simulink model "ModifiedSimulinkModel"  (R2016a)
settings: Solver=ode4  StartTime=0.0  StopTime=200  FixedStep=0.1  RelTol=1e-3
values from neighbouring files (symbols this model uses):
  engineblendfactormap = [0 0 0 0 0 0 0 0 0 0 0 0 ... (420 elements, 21x20)]    [blendfactorvariables.mat]
  motorblendfactormap = [1 1 1 1 1 1 1 1 1 1 1 1 ... (420 elements, 21x20)]    [blendfactorvariables.mat]
  v = [0 5 10 15 20 25 30 35 40 45 50 55 ... (21 elements, 1x21)]    [blendfactorvariables.mat]
  x = [0 1 2 3 4 5 6 7 8 9 10 11 ... (20 elements, 1x20)]    [blendfactorvariables.mat]
undefined symbols (not defined in the file or in its folder): sigbuilder_block
settings Model: Creator=Saumya Trivedi  LastModifiedBy=Saumya Trivedi

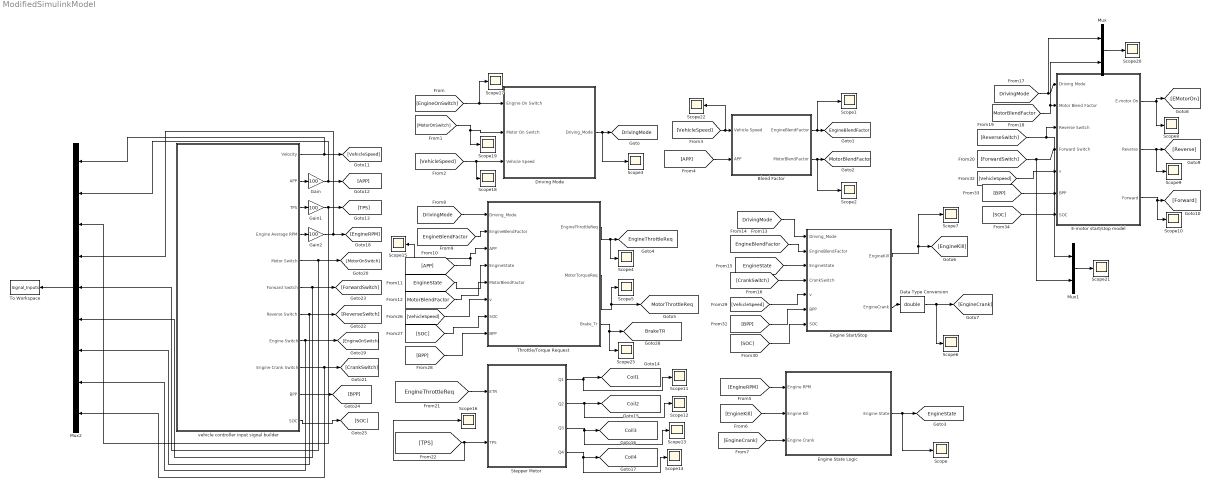
== system ModifiedSimulinkModel ==
  Blend Factor : Subsystem
  Data Type Conversion : DataTypeConversion  OutDataTypeStr=double
  Driving Mode : Subsystem
  E-motor start/stop model : Subsystem
  Engine Start/Stop : Subsystem
  Engine State Logic : Subsystem
  Gain : Gain  Gain=100
  Gain1 : Gain  Gain=100
  Gain2 : Gain  Gain=100
  Mux : Mux  Inputs=2
  Mux1 : Mux  Inputs=2
  Mux2 : Mux  Inputs=9
  Scope{,1..22,25} (24 alike) : Scope
  Stepper Motor : Subsystem
  Throttle/Torque Request : Subsystem
  To Workspace : ToWorkspace  VariableName=Signal_Inputs  SaveFormat=Structure With Time  SampleTime=-1
  vehicle controller input signal builder : Subsystem  Tag=STV Subsys  LoadFcn=sigbuilder_block('load');  StartFcn=sigbuilder_block('start');  StopFcn=sigbuilder_block('stop');  ClipboardFcn=sigbuilder_block('clipboard');  mask(Sigbuilder block){}
      mask help: Create and generate interchangeable groups of signals whose waveforms are piecewise linear.
      mask init:
      | if ~strcmp(get_param(bdroot(gcbh),'SimulationStatus'),'stopped') tuvar = sigbuilder_block('maskInit'); end
      settings: CopyFcn=sigbuilder_block('copy');  DeleteFcn=sigbuilder_block('delete');  ModelCloseFcn=sigbuilder_block('modelClose');  PreSaveFcn=sigbuilder_block('preSave');  PauseFcn=sigbuilder_block('pause')  ContinueFcn=sigbuilder_block('continue')  NameChangeFcn=sigbuilder_block('namechange');  OpenFcn=sigbuilder_block('open',[5.5 33.5 949 407 ]);  CloseFcn=sigbuilder_block('close');
      mask Display: plot(0,0,100,100,[10,10,40,40,10],[80,20,20,80,80],[40,10],[50,50], [40,27,10],[65,72,56],[40,25,25,10],[28,28,43,43]);
  tag scope: BrakeTR=global, Coil1=global, Coil2=global, Coil3=global, Coil4=global, DrivingMode=global, EngineBlendFactor=global, EngineState=global, EngineThrottleReq=global, MotorBlendFactor=global, MotorThrottleReq=global
  wires:
  [EngineOnSwitch] -> Scope17/1, Driving Mode/1(Engine On Switch)
  [MotorOnSwitch] -> Driving Mode/2(Motor On Switch), Scope19/1
  Driving Mode/1(Driving_Mode) -> Scope3/1, [DrivingMode]
  [VehicleSpeed] -> Scope22/1, Blend Factor/1(Vehicle Speed)
  Blend Factor/1(EngineBlendFactor) -> Scope1/1, [EngineBlendFactor]
  Blend Factor/2(MotorBlendFactor) -> Scope2/1, [MotorBlendFactor]
  [EngineRPM] -> Engine State Logic/1(Engine RPM)
  [EngineCrank] -> Engine State Logic/3(Engine Crank)
  [EngineKill] -> Engine State Logic/2(Engine Kill)
  Engine State Logic/1(Engine State) -> Scope/1, [EngineState]
  [DrivingMode] -> Throttle/Torque Request/1(Driving_Mode)
  [EngineBlendFactor] -> Throttle/Torque Request/2(EngineBlendFactor)
  [APP] -> Throttle/Torque Request/3(APP), Scope15/1
  [EngineState] -> Throttle/Torque Request/4(EngineState)
  [MotorBlendFactor] -> Throttle/Torque Request/5(MotorBlendFactor)
  Throttle/Torque Request/1(EngineThrottleReq) -> Scope4/1, [EngineThrottleReq]
  Throttle/Torque Request/2(MotorTorqueReq) -> Scope5/1, [MotorThrottleReq]
  [DrivingMode] -> Engine Start/Stop/1(Driving_Mode)
  [EngineBlendFactor] -> Engine Start/Stop/2(EngineBlendFactor)
  [EngineState] -> Engine Start/Stop/3(EngineState)
  [CrankSwitch] -> Engine Start/Stop/4(CrankSwitch)
  Engine Start/Stop/1(EngineKill) -> Scope7/1, [EngineKill]
  [DrivingMode] -> Mux/1, E-motor start/stop model/1(Driving Mode)
  E-motor start/stop model/1(E-motor On) -> Scope8/1, [EMotorOn]
  E-motor start/stop model/2(Reverse) -> Scope9/1, [Reverse]
  E-motor start/stop model/3(Forward) -> Scope10/1, [Forward]
  [EngineThrottleReq] -> Stepper Motor/1(ETR)
  [TPS] -> Scope16/1, Stepper Motor/2(TPS)
  Stepper Motor/1(Q1) -> [Coil1], Scope11/1
  Stepper Motor/4(Q4) -> Scope14/1, [Coil4]
  Stepper Motor/3(Q3) -> Scope13/1, [Coil3]
  Stepper Motor/2(Q2) -> Scope12/1, [Coil2]
  vehicle controller input signal builder/2(APP) -> Gain/1
  vehicle controller input signal builder/3(TPS) -> Gain1/1
  vehicle controller input signal builder/4(Engine Average RPM) -> Gain2/1
  vehicle controller input signal builder/1(Velocity) -> Mux2/1, [VehicleSpeed]
  Gain/1 -> Mux2/2, [APP]
  Gain1/1 -> Mux2/3, [TPS]
  Gain2/1 -> Mux2/4, [EngineRPM]
  vehicle controller input signal builder/8(Engine Switch) -> Mux2/8, [EngineOnSwitch]
  vehicle controller input signal builder/5(Motor Switch) -> Mux2/5, [MotorOnSwitch]
  vehicle controller input signal builder/9(Engine Crank Switch) -> Mux2/9, [CrankSwitch]
  vehicle controller input signal builder/7(Reverse Switch) -> Mux2/7, [ReverseSwitch]
  vehicle controller input signal builder/6(Forward Switch) -> Mux2/6, [ForwardSwitch]
  vehicle controller input signal builder/10(BPP) -> [BPP]
  [VehicleSpeed] -> Driving Mode/3(Vehicle Speed), Scope18/1
  [MotorBlendFactor] -> Mux/2, E-motor start/stop model/2(Motor Blend Factor)
  [ReverseSwitch] -> Mux1/1, E-motor start/stop model/3(Reverse Switch)
  [ForwardSwitch] -> Mux1/2, E-motor start/stop model/4(Forward Switch)
  Mux/1 -> Scope20/1
  Mux1/1 -> Scope21/1
  Mux2/1 -> To Workspace/1
  Engine Start/Stop/2(EngineCrank) -> Data Type Conversion/1
  Data Type Conversion/1 -> Scope6/1, [EngineCrank]
  [VehicleSpeed] -> Throttle/Torque Request/6(v)
  [SOC] -> Throttle/Torque Request/7(SOC)
  [BPP] -> Throttle/Torque Request/8("BPP ")
  Throttle/Torque Request/3(Brake_Tr) -> Scope25/1, [BrakeTR]
  [BPP] -> Engine Start/Stop/6(BPP)
  [VehicleSpeed] -> Engine Start/Stop/5(v)
  [SOC] -> Engine Start/Stop/7(SOC)
  [SOC] -> E-motor start/stop model/7(SOC)
  [BPP] -> E-motor start/stop model/6(BPP)
  [VehicleSpeed] -> E-motor start/stop model/5(v)
  vehicle controller input signal builder/11(SOC) -> [SOC]
  [APP] -> Blend Factor/2(APP)

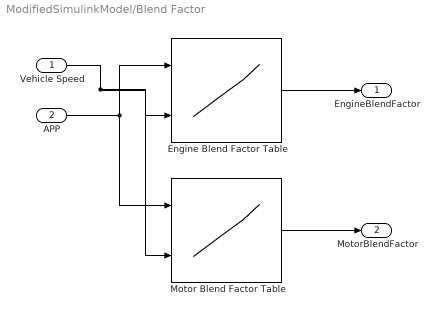
== system ModifiedSimulinkModel/Blend Factor ==
  Vehicle Speed : Inport
  APP : Inport  Port=2
  Engine Blend Factor Table : Lookup_n-D  BreakpointsForDimension1=v  BreakpointsForDimension2=x  Table=engineblendfactormap  InternalRulePriority=Speed  RndMeth=Simplest  InputSameDT=on
  Motor Blend Factor Table : Lookup_n-D  BreakpointsForDimension1=v  BreakpointsForDimension2=x  Table=motorblendfactormap  InternalRulePriority=Speed  RndMeth=Simplest  InputSameDT=on
  EngineBlendFactor : Outport
  MotorBlendFactor : Outport  Port=2
  wires:
  Engine Blend Factor Table/1 -> EngineBlendFactor/1
  APP/1 -> Engine Blend Factor Table/1, Motor Blend Factor Table/1
  Motor Blend Factor Table/1 -> MotorBlendFactor/1
  Vehicle Speed/1 -> Motor Blend Factor Table/2, Engine Blend Factor Table/2

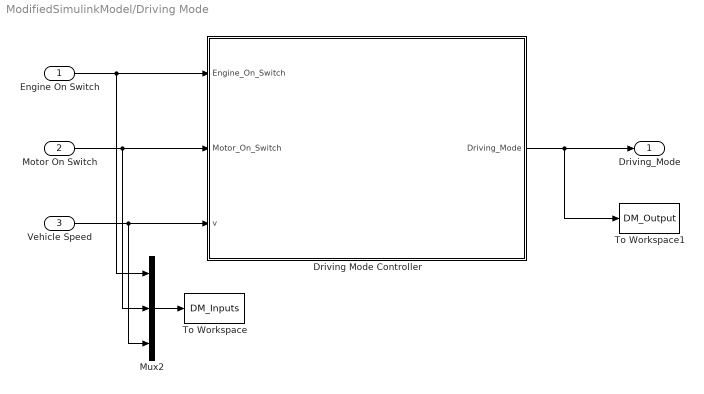
== system ModifiedSimulinkModel/Driving Mode ==
  Engine On Switch : Inport
  Motor On Switch : Inport  Port=2
  Vehicle Speed : Inport  Port=3
  Driving Mode Controller : Stateflow chart  TreatAsAtomicUnit=on
  Mux2 : Mux  Inputs=3
  To Workspace : ToWorkspace  VariableName=DM_Inputs  SaveFormat=Structure With Time  SampleTime=-1
  To Workspace1 : ToWorkspace  VariableName=DM_Output  SaveFormat=Structure With Time  SampleTime=-1
  Driving_Mode : Outport
  wires:
  Engine On Switch/1 -> Mux2/1, Driving Mode Controller/1(Engine_On_Switch)
  Motor On Switch/1 -> Mux2/2, Driving Mode Controller/2(Motor_On_Switch)
  Driving Mode Controller/1(Driving_Mode) -> To Workspace1/1, Driving_Mode/1
  Vehicle Speed/1 -> Mux2/3, Driving Mode Controller/3(v)
  Mux2/1 -> To Workspace/1

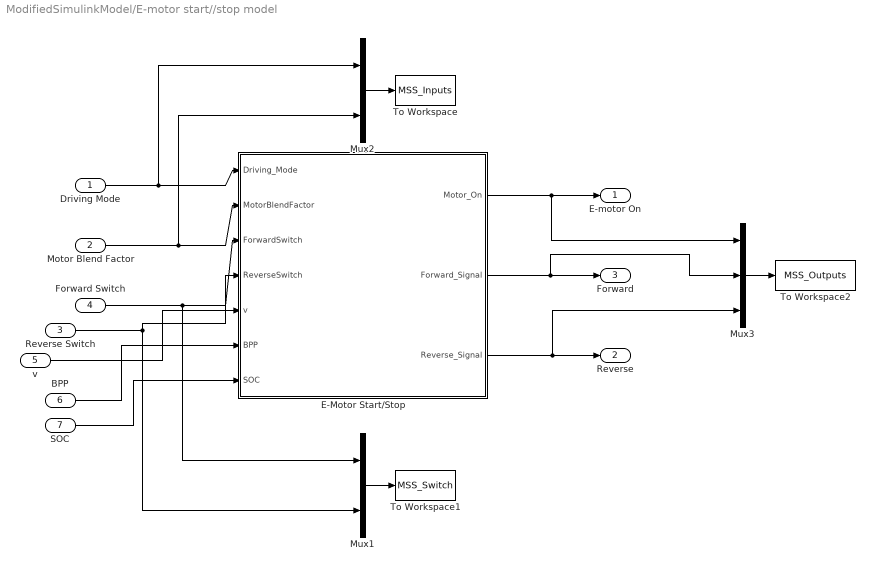
== system ModifiedSimulinkModel/E-motor start//stop model ==
  Driving Mode : Inport
  Motor Blend Factor : Inport  Port=2
  Reverse Switch : Inport  Port=3
  Forward Switch : Inport  Port=4
  v : Inport  Port=5
  BPP : Inport  Port=6
  SOC : Inport  Port=7
  E-Motor Start/Stop : Stateflow chart  TreatAsAtomicUnit=on
  Mux1 : Mux  Inputs=2
  Mux2 : Mux  Inputs=2
  Mux3 : Mux  Inputs=3
  To Workspace : ToWorkspace  VariableName=MSS_Inputs  SaveFormat=Structure With Time  SampleTime=-1
  To Workspace1 : ToWorkspace  VariableName=MSS_Switch  SaveFormat=Structure With Time  SampleTime=-1
  To Workspace2 : ToWorkspace  VariableName=MSS_Outputs  SaveFormat=Structure With Time  SampleTime=-1
  E-motor On : Outport
  Reverse : Outport  Port=2
  Forward : Outport  Port=3
  wires:
  Motor Blend Factor/1 -> Mux2/2, E-Motor Start/Stop/2(MotorBlendFactor)
  Reverse Switch/1 -> E-Motor Start/Stop/4(ReverseSwitch), Mux1/2
  Driving Mode/1 -> Mux2/1, E-Motor Start/Stop/1(Driving_Mode)
  Forward Switch/1 -> Mux1/1, E-Motor Start/Stop/3(ForwardSwitch)
  E-Motor Start/Stop/3(Reverse_Signal) -> Mux3/3, Reverse/1
  E-Motor Start/Stop/1(Motor_On) -> Mux3/1, E-motor On/1
  E-Motor Start/Stop/2(Forward_Signal) -> Mux3/2, Forward/1
  Mux2/1 -> To Workspace/1
  Mux1/1 -> To Workspace1/1
  Mux3/1 -> To Workspace2/1
  SOC/1 -> E-Motor Start/Stop/7(SOC)
  BPP/1 -> E-Motor Start/Stop/6(BPP)
  v/1 -> E-Motor Start/Stop/5(v)

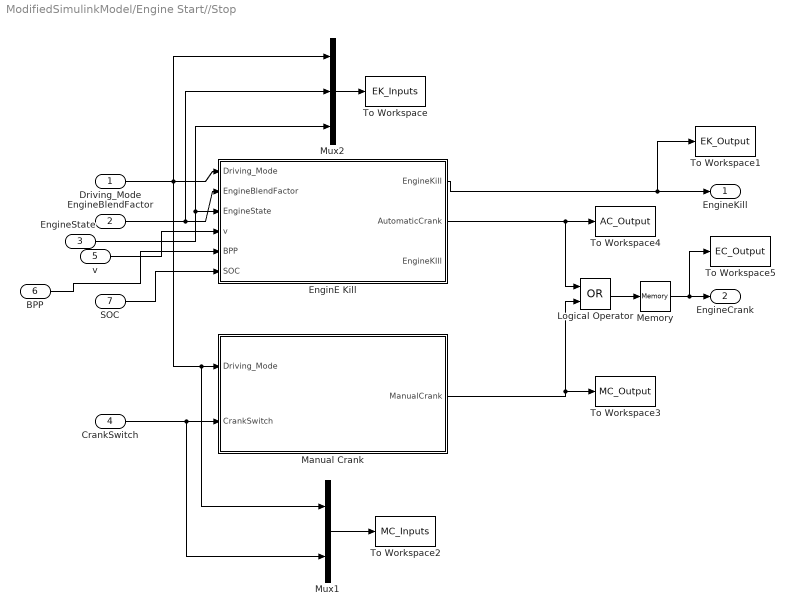
== system ModifiedSimulinkModel/Engine Start//Stop ==
  Driving_Mode : Inport
  EngineBlendFactor : Inport  Port=2
  EngineState : Inport  Port=3
  CrankSwitch : Inport  Port=4
  v : Inport  Port=5
  BPP : Inport  Port=6
  SOC : Inport  Port=7
  EnginE Kill : Stateflow chart  TreatAsAtomicUnit=on
  Logical Operator : Logic  Operator=OR  AllPortsSameDT=off  OutDataTypeStr=boolean
  Manual Crank : Stateflow chart  TreatAsAtomicUnit=on
  Memory : Memory  X0=1
  Mux1 : Mux  Inputs=2
  Mux2 : Mux  Inputs=3
  To Workspace : ToWorkspace  VariableName=EK_Inputs  SaveFormat=Structure With Time  SampleTime=-1
  To Workspace1 : ToWorkspace  VariableName=EK_Output  SaveFormat=Structure With Time  SampleTime=-1
  To Workspace2 : ToWorkspace  VariableName=MC_Inputs  SaveFormat=Structure With Time  SampleTime=-1
  To Workspace3 : ToWorkspace  VariableName=MC_Output  SaveFormat=Structure With Time  SampleTime=-1
  To Workspace4 : ToWorkspace  VariableName=AC_Output  SaveFormat=Structure With Time  SampleTime=-1
  To Workspace5 : ToWorkspace  VariableName=EC_Output  SaveFormat=Structure With Time  SampleTime=-1
  EngineKill : Outport
  EngineCrank : Outport  Port=2
  wires:
  EnginE Kill/2(AutomaticCrank) -> To Workspace4/1, Logical Operator/1
  Logical Operator/1 -> Memory/1
  CrankSwitch/1 -> Mux1/2, Manual Crank/2(CrankSwitch)
  EngineBlendFactor/1 -> Mux2/2, EnginE Kill/2(EngineBlendFactor)
  EngineState/1 -> EnginE Kill/3(EngineState), Mux2/3
  EnginE Kill/1(EngineKill) -> To Workspace1/1, EngineKill/1
  Driving_Mode/1 -> Mux2/1, Mux1/1, Manual Crank/1(Driving_Mode), EnginE Kill/1(Driving_Mode)
  Manual Crank/1(ManualCrank) -> To Workspace3/1, Logical Operator/2
  Mux2/1 -> To Workspace/1
  Mux1/1 -> To Workspace2/1
  SOC/1 -> EnginE Kill/6(SOC)
  BPP/1 -> EnginE Kill/5(BPP)
  v/1 -> EnginE Kill/4(v)
  Memory/1 -> To Workspace5/1, EngineCrank/1

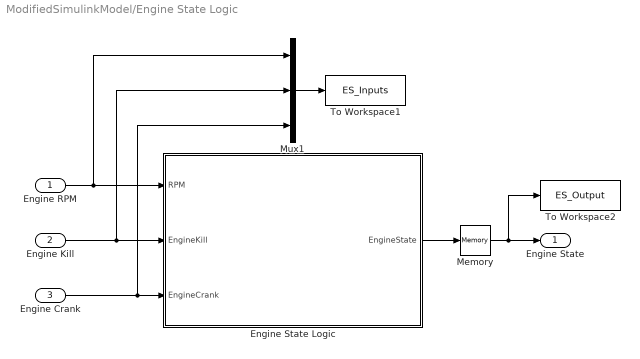
== system ModifiedSimulinkModel/Engine State Logic ==
  Engine RPM : Inport
  Engine Kill : Inport  Port=2
  Engine Crank : Inport  Port=3
  Engine State Logic : Stateflow chart  TreatAsAtomicUnit=on
  Memory : Memory  X0=1
  Mux1 : Mux  Inputs=3
  To Workspace1 : ToWorkspace  VariableName=ES_Inputs  SaveFormat=Structure With Time  SampleTime=-1
  To Workspace2 : ToWorkspace  VariableName=ES_Output  SaveFormat=Structure With Time  SampleTime=-1
  Engine State : Outport
  wires:
  Engine Kill/1 -> Mux1/2, Engine State Logic/2(EngineKill)
  Engine RPM/1 -> Mux1/1, Engine State Logic/1(RPM)
  Engine Crank/1 -> Mux1/3, Engine State Logic/3(EngineCrank)
  Engine State Logic/1(EngineState) -> Memory/1
  Memory/1 -> To Workspace2/1, Engine State/1
  Mux1/1 -> To Workspace1/1

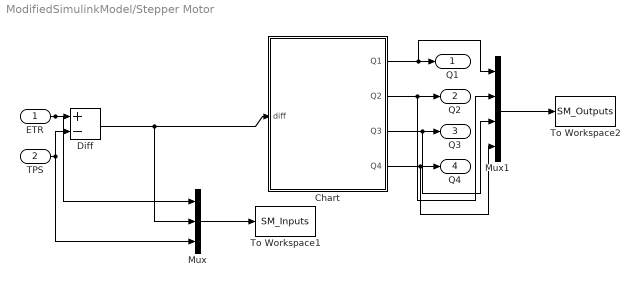
== system ModifiedSimulinkModel/Stepper Motor ==
  ETR : Inport
  TPS : Inport  Port=2
  Chart : Stateflow chart  TreatAsAtomicUnit=on
  Diff : Sum  Inputs=+-
  Mux : Mux  Inputs=3
  Mux1 : Mux
  To Workspace1 : ToWorkspace  VariableName=SM_Inputs  SaveFormat=Structure With Time  SampleTime=-1
  To Workspace2 : ToWorkspace  VariableName=SM_Outputs  SaveFormat=Structure With Time  SampleTime=-1
  Q1 : Outport
  Q2 : Outport  Port=2
  Q3 : Outport  Port=3
  Q4 : Outport  Port=4
  wires:
  TPS/1 -> Mux/3, Diff/2
  Chart/2(Q2) -> Mux1/2, Q2/1
  Chart/3(Q3) -> Mux1/3, Q3/1
  Chart/4(Q4) -> Mux1/4, Q4/1
  Chart/1(Q1) -> Mux1/1, Q1/1
  ETR/1 -> Mux/1, Diff/1
  Diff/1 -> Mux/2, Chart/1(diff)
  Mux/1 -> To Workspace1/1
  Mux1/1 -> To Workspace2/1

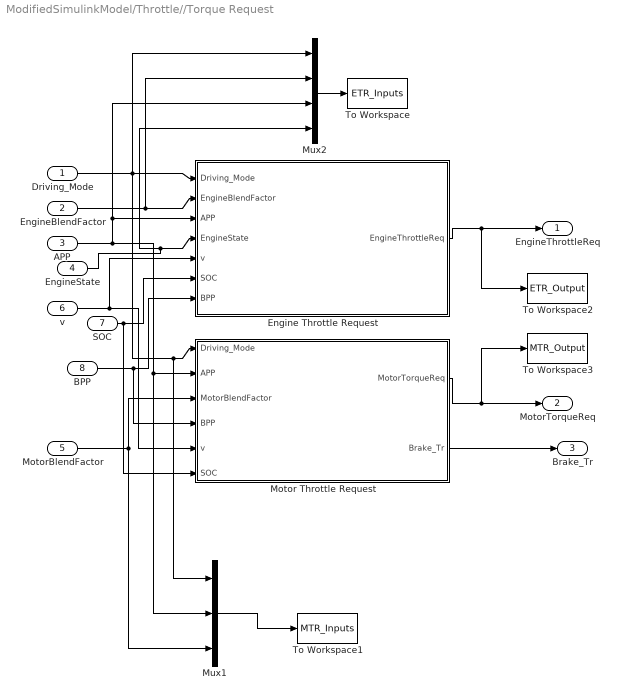
== system ModifiedSimulinkModel/Throttle//Torque Request ==
  Driving_Mode : Inport
  EngineBlendFactor : Inport  Port=2
  APP : Inport  Port=3
  EngineState : Inport  Port=4
  MotorBlendFactor : Inport  Port=5
  v : Inport  Port=6
  SOC : Inport  Port=7
  "BPP " : Inport  Port=8
  Engine Throttle Request : Stateflow chart  TreatAsAtomicUnit=on
  Motor Throttle Request : Stateflow chart  TreatAsAtomicUnit=on
  Mux1 : Mux  Inputs=3
  Mux2 : Mux
  To Workspace : ToWorkspace  VariableName=ETR_Inputs  SaveFormat=Structure With Time  SampleTime=-1
  To Workspace1 : ToWorkspace  VariableName=MTR_Inputs  SaveFormat=Structure With Time  SampleTime=-1
  To Workspace2 : ToWorkspace  VariableName=ETR_Output  SaveFormat=Structure With Time  SampleTime=-1
  To Workspace3 : ToWorkspace  VariableName=MTR_Output  SaveFormat=Structure With Time  SampleTime=-1
  EngineThrottleReq : Outport
  MotorTorqueReq : Outport  Port=2
  Brake_Tr : Outport  Port=3
  wires:
  Driving_Mode/1 -> Mux2/1, Mux1/1, Motor Throttle Request/1(Driving_Mode), Engine Throttle Request/1(Driving_Mode)
  MotorBlendFactor/1 -> Motor Throttle Request/3(MotorBlendFactor), Mux1/3
  Engine Throttle Request/1(EngineThrottleReq) -> To Workspace2/1, EngineThrottleReq/1
  Motor Throttle Request/1(MotorTorqueReq) -> To Workspace3/1, MotorTorqueReq/1
  APP/1 -> Engine Throttle Request/3(APP), Mux2/3, Mux1/2, Motor Throttle Request/2(APP)
  EngineBlendFactor/1 -> Mux2/2, Engine Throttle Request/2(EngineBlendFactor)
  EngineState/1 -> Mux2/4, Engine Throttle Request/4(EngineState)
  Mux2/1 -> To Workspace/1
  Mux1/1 -> To Workspace1/1
  v/1 -> Motor Throttle Request/5(v), Engine Throttle Request/5(v)
  SOC/1 -> Motor Throttle Request/6(SOC), Engine Throttle Request/6(SOC)
  "BPP "/1 -> Motor Throttle Request/4(BPP), Engine Throttle Request/7(BPP)
  Motor Throttle Request/2(Brake_Tr) -> Brake_Tr/1

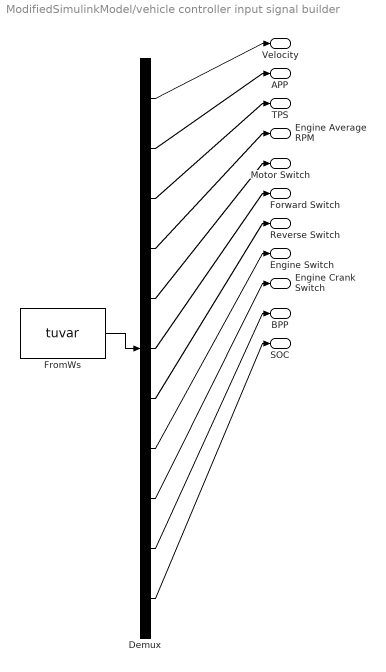
== system ModifiedSimulinkModel/vehicle controller input signal builder ==
  Demux : Demux  Tag=STV Demux  Outputs=11
  FromWs : FromWorkspace  Tag=STV FromWs  VariableName=tuvar  SampleTime=0
      SigBuilderData=|
      | common.afterFinalStr = 'Extrapolate'
      | common.sampleTime = 0
      | dataSet.timeRange = [0 200]
      | dataSet.name = 'Group 1'
      | sbobj.Groups.Name = 'Group 1'
      | sbobj.Groups.Signals(1).Name = 'Velocity'
      | sbobj.Groups.Signals(1).XData = [0 20 30 40 47 50 55 60 100 140 200]
      | sbobj.Groups.Signals(1).YData = [0 0 8 10 0.5 6 6 20 0 20 0]
      | sbobj.Groups.Signals(2).Name = 'APP'
      | sbobj.Groups.Signals(2).XData = [0 20 40 40 50 50 60 60.1 70 100 100 140 140 200]
      | sbobj.Groups.Signals(2).YData = [0 0 0.5 0.2 0.2 0.5 0.5 0 0 0 0.8 0.8 0 0]
      | sbobj.Groups.Signals(3).Name = 'TPS'
      | sbobj.Groups.Signals(3).XData = [0 20 40.1 40.1 50 50.1 60 60.1 100 100 120 120 140 140 200]
      | sbobj.Groups.Signals(3).YData = [0 0 0 0.1 0.1 0.5 0.5 0 0 0.5 0.5 0.8 0.8 0 0]
      | sbobj.Groups.Signals(4).Name = 'Engine Average RPM'
      | sbobj.Groups.Signals(4).XData = [0 20 40.1 44 50 60 70 100 110 120 130 140 140 200]
      | sbobj.Groups.Signals(4).YData = [0 0 0 2 2 8.5 2 2 4 4 10 10 2 0]
      | sbobj.Groups.Signals(5).Name = 'Motor Switch'
      | sbobj.Groups.Signals(5).XData = [0 20 20.1 40 40 180 180 200]
      | sbobj.Groups.Signals(5).YData = [0 0 1 1 0 0 1 1]
      | sbobj.Groups.Signals(6).Name = 'Forward Switch'
      | sbobj.Groups.Signals(6).XData = [0 20 20 40.2 100 100 200]
      | sbobj.Groups.Signals(6).YData = [0 0 1 1 1 0 0]
      | sbobj.Groups.Signals(7).Name = 'Reverse Switch'
      | sbobj.Groups.Signals(7).XData = [0 180 180 200]
      | sbobj.Groups.Signals(7).YData = [0 0 1 1]
      | sbobj.Groups.Signals(8).Name = 'Engine Switch'
      | sbobj.Groups.Signals(8).XData = [0 55 55 60 60 120 120 140 140 200]
      | sbobj.Groups.Signals(8).YData = [0 0 1 1 0 0 1 1 0 0]
      | sbobj.Groups.Signals(9).Name = 'Engine Crank Switch'
      | sbobj.Groups.Signals(9).XData = [0 39.8 40 60 60 100 100 140 140 200]
      | sbobj.Groups.Signals(9).YData = [0 0 1 1 0 0 1 1 0 0.05]
      | sbobj.Groups.Signals(10).Name = 'BPP'
      | sbobj.Groups.Signals(10).XData = [0 60 60.1 100.1 100.1 140 140 200]
      | sbobj.Groups.Signals(10).YData = [0 0 0.5 0.5 0 0 0.2 0.2]
      | sbobj.Groups.Signals(11).Name = 'SOC'
      | sbobj.Groups.Signals(11).XData = [0 10 50 55 70 100 150 200]
      | sbobj.Groups.Signals(11).YData = [1 1 0.29 0.29 0.7 0.7 0.96 0.96]
      | sbobj.Groups.TimeRange = [0 200]
  Velocity : Outport  Tag=STV Outport
  APP : Outport  Tag=STV Outport  Port=2
  TPS : Outport  Tag=STV Outport  Port=3
  Engine Average RPM : Outport  Tag=STV Outport  Port=4
  Motor Switch : Outport  Tag=STV Outport  Port=5
  Forward Switch : Outport  Tag=STV Outport  Port=6
  Reverse Switch : Outport  Tag=STV Outport  Port=7
  Engine Switch : Outport  Tag=STV Outport  Port=8
  Engine Crank Switch : Outport  Tag=STV Outport  Port=9
  BPP : Outport  Tag=STV Outport  Port=10
  SOC : Outport  Tag=STV Outport  Port=11
  wires:
  FromWs/1 -> Demux/1
  Demux/1 -> Velocity/1
  Demux/2 -> APP/1
  Demux/3 -> TPS/1
  Demux/4 -> Engine Average RPM/1
  Demux/5 -> Motor Switch/1
  Demux/6 -> Forward Switch/1
  Demux/7 -> Reverse Switch/1
  Demux/8 -> Engine Switch/1
  Demux/9 -> Engine Crank Switch/1
  Demux/10 -> BPP/1
  Demux/11 -> SOC/1

== stateflow chart ModifiedSimulinkModel/Engine State Logic/Engine State Logic ==
  state EngineCrankState
    en,du:
    EngineState=2;
    EngineCrankTime=temporalCount(sec);
  state EngineOff
    en:EngineState=1;
  state EngineStartFail
    en:EngineState=5;
  state EngineOn
    en:EngineState=4;
  state EngineWarmup
    en,du:
    EngineState=3;
    EngineWarmUpTime=temporalCount(sec);
  (default) -> EngineOff
  EngineOff -> EngineCrankState : [EngineCrank==1 && EngineKill==0]
  EngineStartFail -> EngineOff
  EngineCrankState -> EngineStartFail [order 2] : [RPM<=800&&EngineCrankTime>1]
  EngineCrankState -> EngineWarmup [order 1] : [RPM>800&&EngineCrankTime>0.6]
  EngineOn -> EngineOff : [RPM<50 || EngineKill==1]
  EngineWarmup -> EngineStartFail [order 2] : [RPM<500 && EngineWarmUpTime>1]
  EngineWarmup -> EngineOn [order 1] : [RPM>=500 && EngineWarmUpTime>1]
  data: RPM input; EngineKill input; EngineCrank input; EngineState output; time local; EngineCrankTime local; EngineWarmUpTime local

== stateflow chart ModifiedSimulinkModel/Throttle//Torque Request/Engine Throttle Request ==
  state DWM
    state ElectricSolo
      du:EngineThrottleReq=0;
    state BlendingMode
      state EngineState23
        en,du:
        EngineThrottleReq=7.5;
      state OtherStates
        state ChargeSustain
          state Lowspeed
            du: EngineThrottleReq=APP*(1-EngineBlendFactor);
          state HighSpeed
            en,du:EngineThrottleReq=APP*EngineBlendFactor;
          HighSpeed -> Lowspeed : [v<10]
          Lowspeed -> HighSpeed : [v>=10]
          (default) -> HighSpeed
        state ChargeDepleting
          en,du:
          EngineThrottleReq=APP*EngineBlendFactor;
        ChargeDepleting -> ChargeSustain : [SOC<=0.3]
        ChargeSustain -> ChargeDepleting : [SOC>0.3]
        (default) -> ChargeDepleting
      (default) -> EngineState23 [order 1] : [EngineState==2||EngineState==3]
      EngineState23 -> ? : [EngineState~=2||EngineState~=3]
      (default) -> OtherStates [order 2] : [EngineState~=2||EngineState~=3]
      OtherStates -> ? : [EngineState==2||EngineState==3]
      (default) -> ? [order 1]
    state EngineSole
      du:EngineThrottleReq=APP;
    (junction 3) -> ElectricSolo [order 1] : [Driving_Mode==1]
    (junction 3) -> BlendingMode [order 2] : [Driving_Mode==2]
    BlendingMode -> (junction 3) : [Driving_Mode~=2]
    (junction 3) -> EngineSole [order 3] : [Driving_Mode==3]
    EngineSole -> (junction 3) : [Driving_Mode~=3]
    ElectricSolo -> (junction 3) : [Driving_Mode~=1]
    (default) -> ElectricSolo
  state regeneration
    state Braking [parallel]
      settings: executionOrder=1
      state FrictionBrake
        du:EngineThrottleReq=0;
      state RegenerativeBrake
        du:EngineThrottleReq=0;
      (default) -> FrictionBrake
      FrictionBrake -> RegenerativeBrake : [v>2&&bat_protection_flag==0]
      RegenerativeBrake -> FrictionBrake : [v<=2||bat_protection_flag==1]
    state BatteryProtection [parallel]
      settings: executionOrder=2
      state NoProtection
        en:bat_protection_flag=0;
      state Protection
        en:bat_protection_flag=1;
      (default) -> NoProtection
      NoProtection -> Protection : [SOC>=0.9]
      Protection -> NoProtection : [SOC<0.9]
    (default) -> Braking
  (default) -> DWM
  DWM -> regeneration : [BPP>0]
  regeneration -> DWM : [BPP<=0]
  data: Driving_Mode input; EngineBlendFactor input; APP input; EngineState input; EngineThrottleReq output; v input; SOC input; bat_protection_flag local; BPP input

== stateflow chart ModifiedSimulinkModel/Driving Mode/Driving Mode Controller ==
  state DM
    state EngineSolo
      du:Driving_Mode=3;
    state BlendingMode
      du:Driving_Mode=2;
    state ElectricSolo
      du:Driving_Mode=1;
    EngineSolo -> (junction 14) : [Engine_On_Switch==0||Motor_On_Switch==1]
    (junction 14) -> EngineSolo [order 1] : [Engine_On_Switch==1&&Motor_On_Switch==0&&v<1]
    (junction 14) -> ElectricSolo [order 3] : [Engine_On_Switch==0&&Motor_On_Switch==1&&v<1]
    BlendingMode -> (junction 14) : [Engine_On_Switch==1||Motor_On_Switch==1]
    (junction 14) -> BlendingMode [order 2] : [Engine_On_Switch==0&&Motor_On_Switch==0&&v<1]
    ElectricSolo -> (junction 14) : [Engine_On_Switch==1||Motor_On_Switch==0]
    (default) -> ElectricSolo
  state Nothing
  (default) -> Nothing
  Nothing -> DM : [v<=1]
  DM -> Nothing : [v>1]
  data: Engine_On_Switch input; Motor_On_Switch input; v input; Driving_Mode output

== stateflow chart ModifiedSimulinkModel/Throttle//Torque Request/Motor Throttle Request ==
  state NW
    state EngineSolo
      du:MotorTorqueReq=0;
    state ElectricSolo
      du:MotorTorqueReq=APP;
    state BlendingMode
      state ChargeSustain
        state Lowspeed
          en,du: MotorTorqueReq=APP*(1-MotorBlendFactor);
        state HighSpeed
          en,du:MotorTorqueReq=APP*MotorBlendFactor;
        HighSpeed -> Lowspeed : [v<=10]
        Lowspeed -> HighSpeed : [v>10]
        (default) -> HighSpeed
      state ChargeDepleting
        en,du:
        MotorTorqueReq=APP*MotorBlendFactor;
      ChargeDepleting -> ChargeSustain : [SOC<=0.3]
      ChargeSustain -> ChargeDepleting : [SOC>0.3]
      (default) -> ChargeDepleting
    (junction 5) -> EngineSolo [order 3] : [Driving_Mode==3]
    (junction 5) -> ElectricSolo [order 1] : [Driving_Mode==1]
    ElectricSolo -> (junction 5) : [Driving_Mode~=1]
    EngineSolo -> (junction 5) : [Driving_Mode~=3]
    BlendingMode -> (junction 5) : [Driving_Mode~=2]
    (junction 5) -> BlendingMode [order 2] : [Driving_Mode==2]
    (default) -> ElectricSolo
  state regeneration
    state Braking [parallel]
      settings: executionOrder=1
      state FrictionBrake
        du:MotorTorqueReq=0;
        Brake_Tr=BPP;
      state RegenerativeBrake
        du:MotorTorqueReq=BPP*0.75;
        Brake_Tr=BPP*0.5;
      (default) -> FrictionBrake
      FrictionBrake -> RegenerativeBrake : [v>2&&bat_protection_flag==0]
      RegenerativeBrake -> FrictionBrake : [v<=2||bat_protection_flag==1]
    state BatteryProtection [parallel]
      settings: executionOrder=2
      state NoProtection
        en:bat_protection_flag=0;
      state Protection
        en:bat_protection_flag=1;
      (default) -> NoProtection
      NoProtection -> Protection : [SOC>=0.9]
      Protection -> NoProtection : [SOC<0.9]
    (default) -> Braking
  (default) -> NW
  NW -> regeneration : [BPP>0]
  regeneration -> NW : [BPP<=0]
  data: Driving_Mode input; APP input; MotorBlendFactor input; MotorTorqueReq output; BPP input; v input; Brake_Tr output; bat_protection_flag local; SOC input

== stateflow chart ModifiedSimulinkModel/Engine Start//Stop/EnginE Kill ==
  state EK
    state EngineSolo
      du:EngineKill=0;AutomaticCrank=0;
    state BlendingMode
      state a
        du:EngineKill=0;
        state c
          du:AutomaticCrank=1;
        state c1
          du:AutomaticCrank=0;
        (default) -> c
        c1 -> c : [EngineState==1]
        c -> c1 : [EngineState~=1]
      state b
        du:EngineKill=1;AutomaticCrank=0;
      (default) -> (junction 13)
      (junction 13) -> a [order 1] : [EngineBlendFactor>0.01]
      a -> (junction 13) : [EngineBlendFactor<=0.01]
      b -> (junction 13) : [EngineBlendFactor>0.01]
      (junction 13) -> b [order 2] : [EngineBlendFactor<=0.01]
    state ElectricSolo
      du:EngineKill=1;AutomaticCrank=0;
    (junction 3) -> EngineSolo [order 3] : [Driving_Mode==3]
    EngineSolo -> (junction 3) : [Driving_Mode~=3]
    (junction 3) -> ElectricSolo [order 1] : [Driving_Mode==1]
    (junction 3) -> BlendingMode [order 2] : [Driving_Mode==2]
    BlendingMode -> (junction 3) : [Driving_Mode~=2]
    ElectricSolo -> (junction 3) : [Driving_Mode~=1]
    (default) -> ElectricSolo
  state regeneration
    state Braking [parallel]
      settings: executionOrder=1
      state FrictionBrake
        en:EngineKIll=1;
      state RegenerativeBrake
        en:EngineKill=1;
      (default) -> FrictionBrake
      FrictionBrake -> RegenerativeBrake : [v>2&&bat_protection_flag==0]
      RegenerativeBrake -> FrictionBrake : [v<=2||bat_protection_flag==1]
    state BatteryProtection [parallel]
      settings: executionOrder=2
      state NoProtection
        en:bat_protection_flag=0;
      state Protection
        en:bat_protection_flag=1;
      (default) -> NoProtection
      NoProtection -> Protection : [SOC>=0.9]
      Protection -> NoProtection : [SOC<0.9]
    (default) -> Braking
  (default) -> EK
  EK -> regeneration : [BPP>0]
  regeneration -> EK : [BPP<=0]
  data: Driving_Mode input; EngineBlendFactor input; EngineKill output; EngineState input; AutomaticCrank output; v input; EngineKIll output; bat_protection_flag local; BPP input; SOC input

== stateflow chart ModifiedSimulinkModel/Engine Start//Stop/Manual Crank ==
  state ElectricSolo
    du:ManualCrank=0;
  state EngineSolo
    state On
      du:ManualCrank=1;
    state Off
      du:ManualCrank=0;
    (default) -> (junction 14)
    (junction 14) -> On [order 1] : [CrankSwitch==1]
    (junction 14) -> Off [order 2] : [CrankSwitch==0]
    Off -> (junction 14) : [CrankSwitch~=0]
    On -> (junction 14) : [CrankSwitch~=1]
  state BlendingMode
    du:ManualCrank=0;
  (junction 1) -> EngineSolo [order 3] : [Driving_Mode==3]
  (junction 1) -> ElectricSolo [order 1] : [Driving_Mode==1]
  BlendingMode -> (junction 1) : [Driving_Mode~=2]
  EngineSolo -> (junction 1) : [Driving_Mode~=3]
  ElectricSolo -> (junction 1) : [Driving_Mode~=1]
  (junction 1) -> BlendingMode [order 2] : [Driving_Mode==2]
  (default) -> ElectricSolo
  data: Driving_Mode input; CrankSwitch input; ManualCrank output

== stateflow chart ModifiedSimulinkModel/E-motor start//stop model/E-Motor Start//Stop ==
  state EM
    state BlendingMode
      state B2
        du:Motor_On=0;
        du:Forward_Signal=1;
        du:Reverse_Signal=0;
      state B1
        du:Motor_On=1;
        du:Forward_Signal=1;
        du:Reverse_Signal=0;
      (default) -> (junction 11)
      (junction 11) -> B2 [order 2] : [MotorBlendFactor<=0.01]
      (junction 11) -> B1 [order 1] : [MotorBlendFactor>0.01]
      B1 -> (junction 11) : [MotorBlendFactor<=0.01]
      B2 -> (junction 11) : [MotorBlendFactor>0.01]
    state ElectricSolo
      du:Motor_On=1;
      du:Forward_Signal=ForwardSwitch;
      du:Reverse_Signal=ReverseSwitch;
    state EngineSolo
      du:Motor_On=0;
      du:Forward_Signal=0;
      du:Reverse_Signal=0;
    (default) -> ElectricSolo
    (junction 5) -> BlendingMode [order 2] : [Driving_Mode==2]
    (junction 5) -> ElectricSolo [order 1] : [Driving_Mode==1]
    ElectricSolo -> (junction 5) : [Driving_Mode~=1]
    BlendingMode -> (junction 5) : [Driving_Mode~=2]
    (junction 5) -> EngineSolo [order 3] : [Driving_Mode==3]
    EngineSolo -> (junction 5) : [Driving_Mode~=3]
  state regeneration
    state Braking [parallel]
      settings: executionOrder=1
      state FrictionBrake
        du:Motor_On=0;
        Forward_Signal=1;
        Reverse_Signal=0;
      state RegenerativeBrake
        du:Motor_On=1;
        Forward_Signal=1;
        Reverse_Signal=0;
      (default) -> FrictionBrake
      FrictionBrake -> RegenerativeBrake : [v>2&&bat_protection_flag==0]
      RegenerativeBrake -> FrictionBrake : [v<=2||bat_protection_flag==1]
    state BatteryProtection [parallel]
      settings: executionOrder=2
      state NoProtection
        en:bat_protection_flag=0;
      state Protection
        en:bat_protection_flag=1;
      (default) -> NoProtection
      NoProtection -> Protection : [SOC>=0.9]
      Protection -> NoProtection : [SOC<0.9]
    (default) -> Braking
  (default) -> EM
  EM -> regeneration : [BPP>0]
  regeneration -> EM : [BPP<=0]
  data: Driving_Mode input; MotorBlendFactor input; ForwardSwitch input; ReverseSwitch input; Motor_On output; Forward_Signal output; Reverse_Signal output; v input; bat_protection_flag local; BPP input; SOC input

== stateflow chart ModifiedSimulinkModel/Stepper Motor/Chart ==
  state On
    state Step3
      en:Q1=1;
      Q2=0;
      Q3=0;
      Q4=1;
    state Step4
      en:Q1=0;
      Q2=0;
      Q3=0;
      Q4=1;
    state Step2
      en:Q1=1;
      Q2=0;
      Q3=0;
      Q4=0;
    state Step1
      en:Q1=1;
      Q2=0;
      Q3=1;
      Q4=0;
    state Step5
      en:Q1=0;
      Q2=1;
      Q3=0;
      Q4=1;
    state Step8
      en:Q1=0;
      Q2=0;
      Q3=1;
      Q4=0;
    state Step7
      en:Q1=0;
      Q2=1;
      Q3=1;
      Q4=0;
    state Step6
      en:Q1=0;
      Q2=1;
      Q3=0;
      Q4=0;
    Step4 -> Step3 [order 2] : [after(10,msec)&&diff<=-1]
    Step2 -> Step3 [order 1] : [after(10,msec)&&diff>=1]
    Step3 -> Step4 [order 1] : [after(10,msec)&&diff>=1]
    Step1 -> Step2 [order 1] : [after(10,msec)&&diff>=1]
    Step5 -> Step4 [order 2] : [after(10,msec)&&diff<=-1]
    Step3 -> Step2 [order 2] : [after(10,msec)&&diff<=-1]
    Step4 -> Step5 [order 1] : [after(10,msec)&&diff>=1]
    Step2 -> Step1 [order 2] : [after(10,msec)&&diff<=-1]
    Step6 -> Step5 [order 2] : [after(10,msec)&&diff<=-1]
    (junction 43) -> Step1 [order 2] : [diff>=1]
    Step1 -> Step8 [order 2] : [after(10,msec)&&diff<=-1]
    Step5 -> Step6 [order 1] : [after(10,msec)&&diff>=1]
    Step8 -> Step1 [order 1] : [after(10,msec)&&diff>=1]
    (default) -> (junction 43)
    (junction 43) -> Step8 [order 1] : [diff<=-1]
    Step7 -> Step8 [order 1] : [after(10,msec)&&diff>=1]
    Step8 -> Step7 [order 2] : [after(10,msec)&&diff<=-1]
    Step6 -> Step7 [order 1] : [after(10,msec)&&diff>=1]
    Step7 -> Step6 [order 2] : [after(10,msec)&&diff<=-1]
  state Off
    en:Q1=0;
    Q2=0;
    Q3=0;
    Q4=0;
  On -> Off : [diff>=-1&&diff<=1]
  Off -> On : [diff>1||diff<-1]
  (default) -> Off
  data: diff input; Q1 output; Q2 output; Q3 output; Q4 output
